simulink model "b_1_tsmds_step"  (R2020b)
settings: Solver=ode45  StartTime=0.0  StopTime=10.0  MaxStep=0.002  RelTol=1e-3
undefined symbols (not defined in the file): c1, c2, k1, k2, m1, m2
settings Model: Creator=rajag  LastModifiedBy=rajag

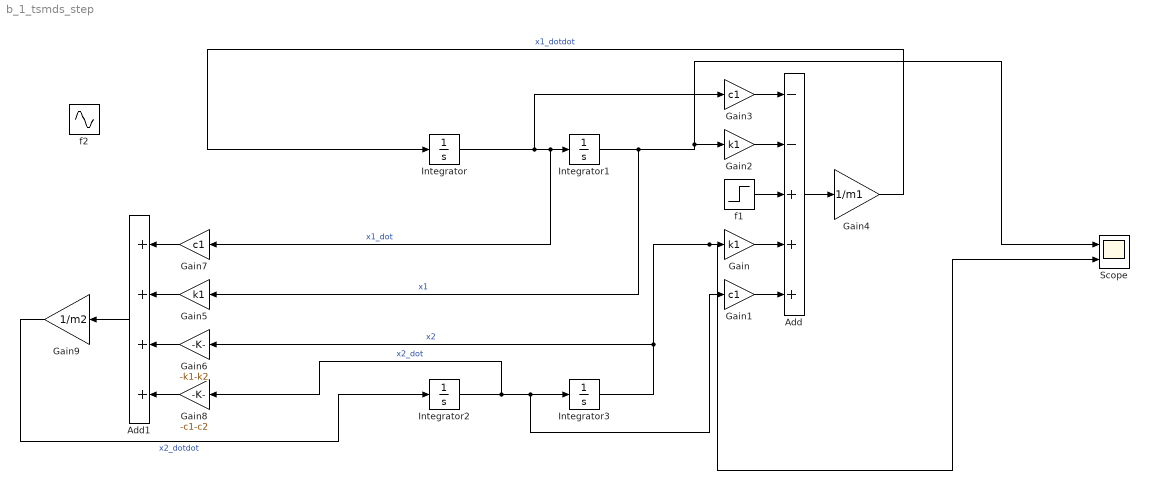
== system b_1_tsmds_step ==
  Add : Sum  Inputs=--+++
  Add1 : Sum  Inputs=++++
  Gain : Gain  Gain=k1
  Gain1 : Gain  Gain=c1
  Gain2 : Gain  Gain=k1
  Gain3 : Gain  Gain=c1
  Gain4 : Gain  Gain=1/m1
  Gain5 : Gain  Gain=k1
  Gain6 : Gain  Gain=-k1-k2
  Gain7 : Gain  Gain=c1
  Gain8 : Gain  Gain=-c1-c2
  Gain9 : Gain  Gain=1/m2
  Integrator{,1..3} (4 alike) : Integrator
  Scope : Scope  NumInputPorts=2
  f1 : Step  After=5  SampleTime=0
  f2 : Sin  Amplitude=3  Frequency=10  SampleTime=0
  wires:
  Integrator/1 -> Gain3/1, Gain7/1, Integrator1/1  "x1_dot"
  Gain4/1 -> Integrator/1  "x1_dotdot"
  Integrator1/1 -> Gain5/1, Scope/1, Gain2/1  "x1"
  Integrator3/1 -> Gain6/1, Scope/2, Gain/1  "x2"
  Integrator2/1 -> Gain8/1, Gain1/1, Integrator3/1  "x2_dot"
  Gain9/1 -> Integrator2/1  "x2_dotdot"
  Gain3/1 -> Add/1
  Gain2/1 -> Add/2
  Gain/1 -> Add/4
  Gain1/1 -> Add/5
  Add/1 -> Gain4/1
  Gain7/1 -> Add1/1
  Gain5/1 -> Add1/2
  Gain6/1 -> Add1/3
  Gain8/1 -> Add1/4
  Add1/1 -> Gain9/1
  f1/1 -> Add/3
